simulink model "adc_demo"  (R2014a)
settings: Solver=ode45  StartTime=0.0  StopTime=1  RelTol=1e-3
libraries: simulink_extras x1
settings Model: Creator=rcheng  LastModifiedBy=rodralez
settings DataIOCC: SignalLoggingSaveFormat=ModelDataLogs
settings OptimizationCC: ExpressionDepthLimit=2147483647  InitFltsAndDblsToZero=on
settings DebuggingCC: UnderspecifiedInitializationDetection=Classic  FcnCallInpInsideContextMsg=UseLocalSettings  StateNameClashWarn=warning
settings GRTTargetCC: CombineOutputUpdateFcns=off  GRTInterface=on

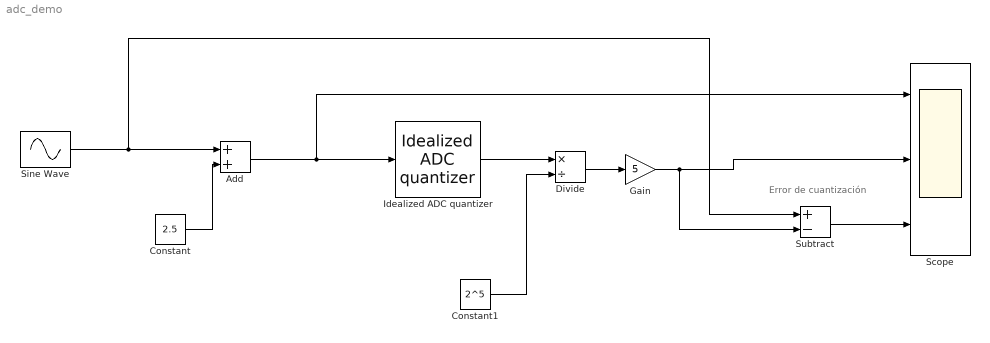
== system adc_demo ==
  note: Error de cuantización
  Add : Sum
  Constant : Constant  Value=2.5
  Constant1 : Constant  Value=2^5
  Divide : Product  Inputs=*/
  Gain : Gain  Gain=5
  Idealized ADC quantizer : simulink_extras/Additional Discrete/Idealized ADC quantizer  NumberOfConverterBits=5  Vmin=0  Vmax=5  OutputDataType=double  OutputNegativeValues=off
  Scope : Scope  NumInputPorts=3
      settings: ShowLegends=on  YMin=-5~-5~-5  YMax=5~5~5
  Sine Wave : Sin  Amplitude=2  Frequency=2*pi*2  SampleTime=1/10000
  Subtract : Sum  Inputs=+-
  wires:
  Sine Wave/1 -> Add/1, Subtract/1
  Subtract/1 -> Scope/3
  Add/1 -> Scope/1, Idealized ADC quantizer/1
  Constant/1 -> Add/2
  Idealized ADC quantizer/1 -> Divide/1
  Constant1/1 -> Divide/2
  Divide/1 -> Gain/1
  Gain/1 -> Subtract/2, Scope/2
